simulink model "DeadBlock1"  (Simulink 7.9)
settings: Solver=ode45  StartTime=0.0  StopTime=10.0  RelTol=1e-3
settings Model: Creator=boakes  LastModifiedBy=boakes

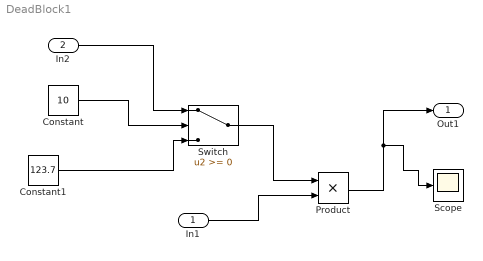
== system DeadBlock1 ==
  In1 : Inport
  In2 : Inport  Port=2
  Constant : Constant  Value=10
  Constant1 : Constant  Value=123.7
  Product : Product  RndMeth=Zero
  Scope : Scope
  Switch : Switch
  Out1 : Outport
  wires:
  In1/1 -> Product/2
  Product/1 -> Out1/1, Scope/1
  Switch/1 -> Product/1
  Constant/1 -> Switch/2
  In2/1 -> Switch/1
  Constant1/1 -> Switch/3
